simulink model "sedemo_rsim_resource_alloc"  (Simulink 7.5)
settings: Solver=VariableStepDiscrete  StartTime=0.0  StopTime=1000  MaxStep=inf  RelTol=1e-3
PreLoadFcn:
  | TrialPoolSize = 3;
undefined symbols (not defined in the file or in its folder): des_subsystemblock, des_subsysteminport, des_subsystemoutport, des_subsystemsupportblock
libraries: simeventssink1 x4, simeventsrouting1 x4, simeventsgenerators1 x3, simeventsqueue1 x2, simeventstranslate1 x2, simeventsserver1 x2, simeventsentitymanage1 x2, simeventsattributes2 x1, simeventsprobes1 x1, simeventsinfo x1
CloseFcn:
  | clear TrialPoolSize;
settings Model: Creator=The MathWorks Inc.  TunableVars=TrialPoolSize  TunableVarsStorageClass=Auto
settings DataIOCC: SaveOutput=off  SaveTime=off
settings OptimizationCC: InlineParams=on
settings DebuggingCC: AlgebraicLoopMsg=error  SolverPrmCheckMsg=none  StrictBusMsg=Warning
settings HardwareCC: TargetEndianess=LittleEndian  TargetHWDeviceType=MATLAB Host  ProdEqTarget=off
settings RTWCC: SystemTargetFile=rsim.tlc  TemplateMakefile=rsim_default_tmf  Description=Rapid Simulation Target  RTWVerbose=off  ProcessScript=rsim_make_rtw_hook
settings RSimTargetCC: TargetFunctionLibrary=ANSI_C  ERTMultiwordTypeDef=System defined  ERTCodeCoverageTool=None  ERTMultiwordLength=256  IsPILTarget=off  EnableShiftOperators=on  PortableWordSizes=off
settings SimEventsCC: propDiagAttribOutput=1  propDiagFcnCallOutput=1  propDiagStatOutput=0

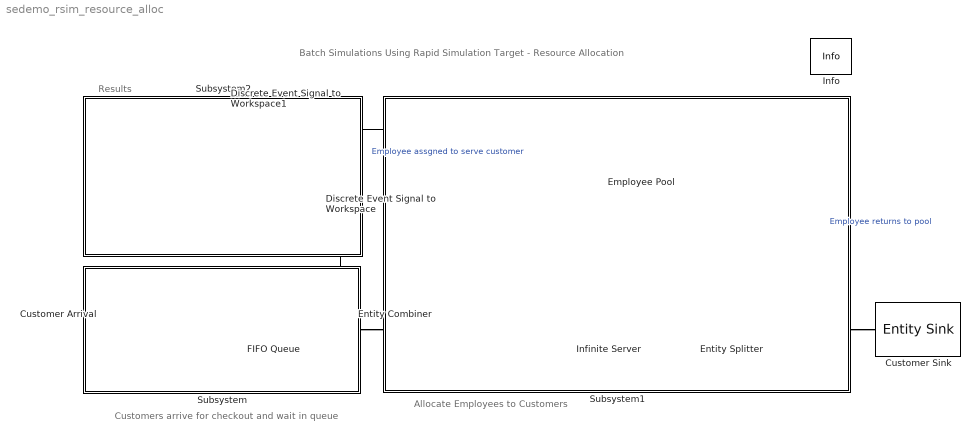
== system sedemo_rsim_resource_alloc ==
  note: Batch Simulations Using Rapid Simulation Target - Resource Allocation
  note: Customers arrive for checkout and wait in queue
  note: Allocate Employees to Customers
  note: Results
  Customer Arrival : Subsystem
  Customer Sink : simeventssink1/Entity Sink  Priority=1  SystemSampleTime=-1  AvailableForArrivals=on  StatNumberArrived=Off
  Discrete Event Signal to Workspace : simeventssink1/Discrete Event Signal to Workspace  SystemSampleTime=-1  VariableName=customer_wait  SaveFormat=Structure With Time  IsMonitorOnly=off  IsRecordIC=off
  Discrete Event Signal to Workspace1 : simeventssink1/Discrete Event Signal to Workspace  SystemSampleTime=-1  VariableName=employee_idle  SaveFormat=Structure With Time  IsMonitorOnly=off  IsRecordIC=off
  Employee Pool : Subsystem  mask{PoolSize=TrialPoolSize}
      mask prompts: PoolSize "Size of Employee Pool"
  Entity Combiner : simeventsentitymanage1/Entity Combiner  Priority=1  SystemSampleTime=-1  NumberInputPorts=2  RetainComponentEntities=on  AttributeAccessibility=on  TimerAccessibility=on  AttributeCopied=on  TimerCopied=on  StatNumberDeparted=Off  EvaluatedNumPorts=2
      settings: AttributesFormatString=Employee assigned to\nserve the customer
  Entity Splitter : simeventsentitymanage1/Entity Splitter  Priority=1  SystemSampleTime=-1  NumberOutputPorts=2  SplitEntityWhen=All entity output ports are not blocked  OutputPortPrecedence=OUT1 port  InitialSeed=56789  ActionUponPortMismatch=Continue  ActionUponBlocking=Discard entity  StatNumberArrived=Off  StatNumberDeparted=Off  EvaluatedNumPorts=2
      settings: AttributesFormatString=Service Completed
  FIFO Queue : simeventsqueue1/FIFO Queue  Priority=1  SystemSampleTime=-1  Capacity=25  EnableTOPort=off  StatNumberDeparted=Off  StatNumberInBlock=Off  StatPendingEntity=Off  StatAverageWait=On  StatAverageQueueLength=Off  StatNumberTimedout=Off
      settings: AttributesFormatString=Customer queue
  Infinite Server : simeventsserver1/Infinite Server  Priority=1  SystemSampleTime=-1  ServiceTimeFrom=Attribute  ServiceTime=1  AttributeName=ServiceTime  PriorityServiceCompletion=500  EnableTOPort=off  StatNumberDeparted=Off  StatNumberInBlock=Off  StatPendingEntity=Off  StatNumberPending=Off  StatAverageWait=Off  StatNumberTimedout=Off
      settings: AttributesFormatString=Employee serves\nthe customer
  Info : simeventsinfo/Info  SystemSampleTime=-1
  Subsystem : Subsystem
      mask Display: disp('')
  Subsystem1 : Subsystem
      mask Display: disp('')
  Subsystem2 : Subsystem
      mask Display: disp('')
  wires:
  FIFO Queue/1 -> Discrete Event Signal to Workspace/1
  Employee Pool/1(idle) -> Discrete Event Signal to Workspace1/1
  connections:
  Customer Arrival/RConn1 -- FIFO Queue/LConn1
  FIFO Queue/RConn1 -- Entity Combiner/LConn2
  Entity Combiner/RConn1 -- Infinite Server/LConn1
  Infinite Server/RConn1 -- Entity Splitter/LConn1
  Entity Splitter/RConn2 -- Customer Sink/LConn1
  Employee Pool/RConn1 -- Entity Combiner/LConn1  "Employee assgned to serve customer"
  Entity Splitter/RConn1 -- Employee Pool/LConn1  "Employee returns to pool"

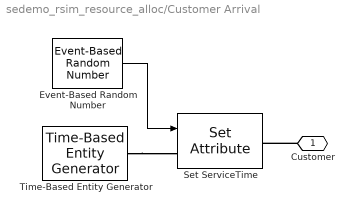
== system sedemo_rsim_resource_alloc/Customer Arrival ==
  Event-Based Random Number : simeventsgenerators1/Signal Generators/Event-Based Random Number  SystemSampleTime=-1  distribution=Uniform  meanExp=2  minUnif=2  maxUnif=10  pOneBern=0.25  pSuccessBino=0.5  numTrialBino=1  meanNorm=0  stdNorm=1  minTri=1  maxTri=3  modeTri=2  thresholdLogn=0  scaleLogn=1  shapeLogn=1  pSuccessGeo=0.5  meanPoiss=1  thresholdLogl=0  scaleLogl=1  thresholdGam=0  scaleGam=1  shapeGam=1  minBeta=0  maxBeta=1  shape1Beta=1  shape2Beta=1  minUnid=0  maxUnid=1  numValueUnid=2  thresholdWbl=0  scaleWbl=1  shapeWbl=1  valueVecCont=[0 1]  cdfVecCont=[0 1]  valueVecDisc=[0 1]  probVecDisc=[0.5 0.5]  seed=6723510  IsProcessed=on  isConnected=1
  Set ServiceTime : simeventsattributes2/Set Attribute  Priority=1  DialogController=des_ddg_create  DialogControllerArgs=DataTag1  SystemSampleTime=-1  AttributeFrom=Signal port  AttributeName=ServiceTime  AttributeTreatAsVector=1  AttributeValue=1  AttributeCreate=on  StatNumberDeparted=Off  EvaluatedAttributeValue={[]}
  Time-Based Entity Generator : simeventsgenerators1/Entity Generators/Time-Based Entity Generator  Priority=1  DialogController=des_ddg_create  DialogControllerArgs=DataTag3  SystemSampleTime=-1  GenerateEntitiesUpon=Intergeneration time from dialog  Distribution=Exponential  Minimum=0  Maximum=1  Mean=1  InitialSeed=6726727  Period=1  PriorityEntityGeneration=300  GenerateEntityAtSimulationStart=on  ResponseWhenBlocked=Pause generation  ResponseWhenUnblocked=Immediate restart  EntityType=Blank  StatNumberDeparted=Off  StatPendingEntity=Off  StatAverageIntergenerationTime=Off
  Customer : PMIOPort  Port=1  Side=Right
  wires:
  Event-Based Random Number/1 -> Set ServiceTime/1
  connections:
  Time-Based Entity Generator/RConn1 -- Set ServiceTime/LConn1
  Customer/RConn1 -- Set ServiceTime/RConn1

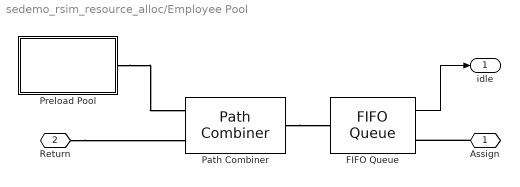
== system sedemo_rsim_resource_alloc/Employee Pool ==
  FIFO Queue : simeventsqueue1/FIFO Queue  Priority=1  SystemSampleTime=-1  Capacity=25  EnableTOPort=off  StatNumberDeparted=Off  StatNumberInBlock=Off  StatPendingEntity=Off  StatAverageWait=On  StatAverageQueueLength=Off  StatNumberTimedout=Off
      settings: AttributesFormatString=Employee Pool
  Path Combiner : simeventsrouting1/Path Combiner  Priority=1  SystemSampleTime=-1  NumberInputPorts=2  InputPortPrecedence=IN1 port  InitialSeed=45675  SpecifyEventPriority=off  PriorityPathCombinerPortPrecedenceSelection=4100  StatNumberDeparted=Off  StatLastArrivalPort=Off  EvaluatedNumPorts=2
  Preload Pool : Subsystem
  Assign : PMIOPort  Port=1  Side=Right
  Return : PMIOPort  Port=2  Side=Left
  idle : Outport
  wires:
  FIFO Queue/1 -> idle/1
  connections:
  Path Combiner/RConn1 -- FIFO Queue/LConn1
  Assign/RConn1 -- FIFO Queue/RConn1
  Return/RConn1 -- Path Combiner/LConn2
  Preload Pool/RConn1 -- Path Combiner/LConn1

== system sedemo_rsim_resource_alloc/Subsystem ==

== system sedemo_rsim_resource_alloc/Subsystem1 ==

== system sedemo_rsim_resource_alloc/Subsystem2 ==

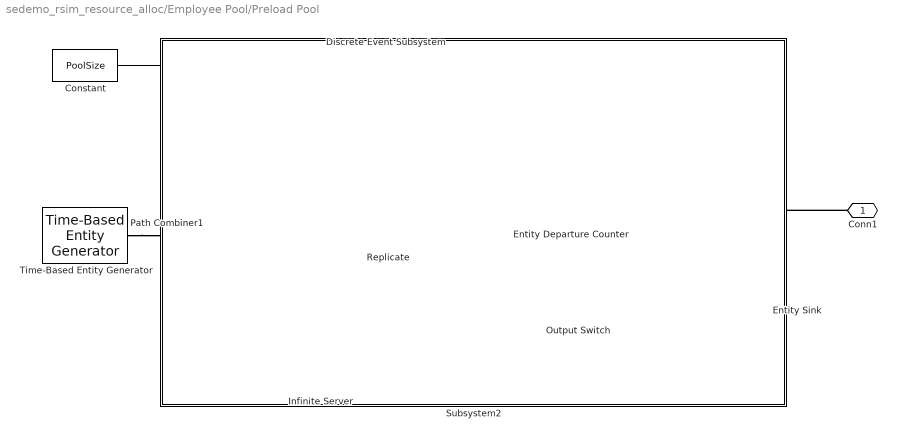
== system sedemo_rsim_resource_alloc/Employee Pool/Preload Pool ==
  Constant : Constant  Value=PoolSize  OutDataType=fixdt(1, 16)  OutScaling=2^0
  Discrete Event Subsystem : Subsystem  LoadFcn=des_subsystemblock(gcb, 'load');  InitFcn=des_subsystemblock(gcb, 'init');  StartFcn=des_subsystemblock(gcb, 'start');  StopFcn=des_subsystemblock(gcb, 'stop');
      settings: CopyFcn=des_subsystemblock(gcb, 'copy');  DeleteFcn=des_subsystemblock(gcb, 'delete');  UndoDeleteFcn=des_subsystemblock(gcb, 'undodelete');  ModelCloseFcn=des_subsystemblock(gcb, 'modelclose');  PreSaveFcn=des_subsystemblock(gcb, 'presave');  NameChangeFcn=des_subsystemblock(gcb, 'namechange');  OpenFcn=des_subsystemblock(gcb, 'open');  ParentCloseFcn=des_subsystemblock(gcb, 'parentclose');  ErrorFcn=des_subsystemerror
      mask Type: Discrete Event Subsystem
      mask Help: helpview(simeventsbhelp);
  Entity Departure Counter : simeventsprobes1/Entity Departure Counter  Priority=1  SystemSampleTime=-1  NumberDepartedToSignal=On  NumberDepartedToAttribute=Off  NumberDepartedAttributeName=Count  CreateAttribute=on  CounterResetTypeOption=Trigger from port tr  CounterResetEdgeOption=Rising  SpecifyEventPriority=on  PriorityEntityCounterReset=1
  Entity Sink : simeventssink1/Entity Sink  Priority=1  SystemSampleTime=-1  AvailableForArrivals=on  StatNumberArrived=Off
  Infinite Server : simeventsserver1/Infinite Server  Priority=1  SystemSampleTime=-1  ServiceTimeFrom=Dialog  ServiceTime=0  AttributeName=ServiceTime  PriorityServiceCompletion=10  EnableTOPort=off  StatNumberDeparted=Off  StatNumberInBlock=Off  StatPendingEntity=Off  StatNumberPending=Off  StatAverageWait=Off  StatNumberTimedout=Off
  Output Switch : simeventsrouting1/Output Switch  Priority=1  SystemSampleTime=-1  NumberOutputPorts=2  SwitchingCriterion=From signal port p  InitialSeed=34567  AttributeName=Attribute1  InitialConditionsOpt=on  InitialConditions=1  EntityBufferOpt=on  SpecifyEventPriority=off  PriorityOutputSwitchSelectPort=4100  TimeoutPortOpt=off  StatNumberDeparted=Off  StatNumberTimedOut=Off  StatPendingEntity=Off  StatLastDeparturePort=Off  EvaluatedNumPorts=2
  Path Combiner1 : simeventsrouting1/Path Combiner  Priority=1  SystemSampleTime=-1  NumberInputPorts=2  InputPortPrecedence=IN1 port  InitialSeed=45675  SpecifyEventPriority=off  PriorityPathCombinerPortPrecedenceSelection=4100  StatNumberDeparted=Off  StatLastArrivalPort=Off  EvaluatedNumPorts=2
  Replicate : simeventsrouting1/Replicate  Priority=1  SystemSampleTime=-1  NumberOutputPorts=2  ReplicateEntityWhen=All entity output ports are not blocked  OutputPortPrecedence=OUT1 port  InitialSeed=56789  ActionUponBlocking=Discard entity  StatNumberArrived=Off  StatNumberDeparted=Off  EvaluatedNumPorts=2
  Subsystem2 : Subsystem
      mask Display: disp('')
  Time-Based Entity Generator : simeventsgenerators1/Entity Generators/Time-Based Entity Generator  Priority=1  DialogController=des_ddg_create  DialogControllerArgs=DataTag24  SystemSampleTime=-1  GenerateEntitiesUpon=Intergeneration time from dialog  Distribution=Constant  Minimum=0  Maximum=1  Mean=2  InitialSeed=6726727  Period=1e5  PriorityEntityGeneration=10  GenerateEntityAtSimulationStart=on  ResponseWhenBlocked=Pause generation  ResponseWhenUnblocked=Immediate restart  EntityType=Blank  StatNumberDeparted=Off  StatPendingEntity=Off  StatAverageIntergenerationTime=Off
  Conn1 : PMIOPort  Port=1  Side=Right
  wires:
  Entity Departure Counter/1 -> Discrete Event Subsystem/2(Din1)
  Discrete Event Subsystem/2(Dout1) -> Entity Departure Counter/1
  Discrete Event Subsystem/1(Dout) -> Output Switch/1
  Constant/1 -> Discrete Event Subsystem/1(Din)
  connections:
  Replicate/RConn1 -- Entity Departure Counter/LConn1
  Output Switch/RConn2 -- Entity Sink/LConn1
  Output Switch/RConn1 -- Infinite Server/LConn1
  Infinite Server/RConn1 -- Path Combiner1/LConn1
  Replicate/RConn2 -- Output Switch/LConn1
  Time-Based Entity Generator/RConn1 -- Path Combiner1/LConn2
  Path Combiner1/RConn1 -- Replicate/LConn1
  Conn1/RConn1 -- Entity Departure Counter/RConn1

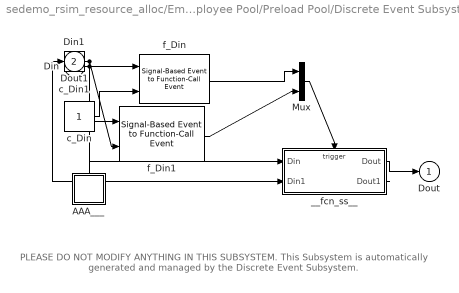
== system sedemo_rsim_resource_alloc/Employee Pool/Preload Pool/Discrete Event Subsystem ==
  note: PLEASE DO NOT MODIFY ANYTHING IN THIS SUBSYSTEM.
      | This Subsystem is automatically generated and
      | managed by the Discrete Event Subsystem.
  Din : Inport  DataType=double  OutDataType=sfix(16)  OutScaling=2^0  OutDataTypeStr=double
  Din1 : Inport  Port=2  DataType=double  OutDataTypeStr=double
  AAA___ : Subsystem  LoadFcn=des_subsystemsupportblock(gcb, 'load');  InitFcn=des_subsystemsupportblock(gcb, 'init');  StartFcn=des_subsystemsupportblock(gcb, 'start');  StopFcn=des_subsystemsupportblock(gcb, 'stop');
      settings: CopyFcn=des_subsystemsupportblock(gcb, 'copy');  DeleteFcn=des_subsystemsupportblock(gcb, 'delete');  UndoDeleteFcn=des_subsystemsupportblock(gcb, 'undodelete');  ModelCloseFcn=des_subsystemsupportblock(gcb, 'modelclose');  PreSaveFcn=des_subsystemsupportblock(gcb, 'presave');  NameChangeFcn=des_subsystemsupportblock(gcb, 'namechange');  OpenFcn=des_subsystemsupportblock(gcb, 'open');  ParentCloseFcn=des_subsystemsupportblock(gcb, 'parentclose');
  Mux : Mux  Inputs=2
  __fcn_ss__ : Subsystem  TreatAsAtomicUnit=on
      settings: PropExecContextOutsideSubsystem=on
  c_Din : Constant  OutDataType=sfix(16)  OutScaling=2^0
  c_Din1 : Constant
  f_Din : simeventstranslate1/Signal-Based Event to Function-Call Event  Priority=1  SystemSampleTime=-1  GenerateFunctionCallUpon=Sample time hit from port ts  SignalEdgeOption=Rising  EnableE1Port=on  EnableF2Port=off  EnableE2Port=off  SpecifyEventPriority=off  PriorityFunctionCall=20  FunctionCallDelayFrom=Dialog  DelayFunctionCall=0  StatNumberF1Calls=Off  StatNumberF2Calls=Off  MaskBlockType=DESS_EVENT_PORT
  f_Din1 : simeventstranslate1/Signal-Based Event to Function-Call Event  Priority=1  SystemSampleTime=-1  GenerateFunctionCallUpon=Sample time hit from port ts  SignalEdgeOption=Rising  EnableE1Port=on  EnableF2Port=off  EnableE2Port=off  SpecifyEventPriority=off  PriorityFunctionCall=20  FunctionCallDelayFrom=Dialog  DelayFunctionCall=0  StatNumberF1Calls=Off  StatNumberF2Calls=Off  MaskBlockType=DESS_EVENT_PORT
  Dout : Outport  OutDataType=sfix(16)  OutScaling=2^0
  Dout1 : Outport  Port=2
  wires:
  __fcn_ss__/1(Dout) -> Dout/1
  f_Din/1 -> Mux/1
  c_Din/1 -> f_Din/2
  Mux/1 -> __fcn_ss__/Trigger
  f_Din1/1 -> Mux/2
  c_Din1/1 -> f_Din1/2
  __fcn_ss__/2(Dout1) -> Dout1/1
  Din/1 -> f_Din/1, __fcn_ss__/1(Din)
  Din1/1 -> f_Din1/1, __fcn_ss__/2(Din1)

== system sedemo_rsim_resource_alloc/Employee Pool/Preload Pool/Subsystem2 ==

== system sedemo_rsim_resource_alloc/Employee Pool/Preload Pool/Discrete Event Subsystem/AAA___ ==

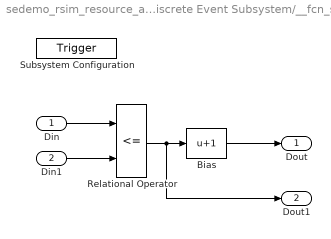
== system sedemo_rsim_resource_alloc/Employee Pool/Preload Pool/Discrete Event Subsystem/__fcn_ss__ ==
  Din : Inport  LoadFcn=des_subsysteminport(gcb, 'load');  InitFcn=des_subsysteminport(gcb, 'init');  StartFcn=des_subsysteminport(gcb, 'start');  StopFcn=des_subsysteminport(gcb, 'stop');  OutDataType=sfix(16)  OutScaling=2^0  mask(Discrete Event Inport){PermitSubsystemEvents=on, TypeOfEvent=Sample time hit, SignalEdgeOption=Rising, SpecifyEventPriority=off, PrioritySubsystemEvent=20}
      mask prompts: PermitSubsystemEvents "Execute subsystem upon signal-based events"; TypeOfEvent "Type of signal-based event:"; SignalEdgeOption "Type of change in signal value:"; SpecifyEventPriority "Resolve simultaneous signal updates according to event priority"; PrioritySubsystemEvent "Event priority:"
      mask help: Input port for a Discrete Event Subsystem block. This block can conditionally execute the subsystem upon signal-based events that meet specified criteria.
      mask init:
      | des_subsystemmask(gcb, 'init','apply')
      settings: CopyFcn=des_subsysteminport(gcb, 'copy');  DeleteFcn=des_subsysteminport(gcb, 'delete');  UndoDeleteFcn=des_subsysteminport(gcb, 'undodelete');  ModelCloseFcn=des_subsysteminport(gcb, 'modelclose');  PreSaveFcn=des_subsysteminport(gcb, 'presave');  NameChangeFcn=des_subsysteminport(gcb, 'namechange');  ParentCloseFcn=des_subsysteminport(gcb, 'parentclose');
      mask Help: helpview(simeventsbhelp);
      mask StyleString: checkbox,popup(Change in signal|Trigger|Sample time hit),popup(Rising|Falling|Either),checkbox,edit
      mask CallbackString: des_subsystemmask(gcb, 'cbPermitSubsystemEvents', 'noapply');|des_subsystemmask(gcb,'cbTypeOfEvent','noapply');||des_subsystemmask(gcb, 'cbSpecifyEventPriority', 'noapply');|
  Din1 : Inport  LoadFcn=des_subsysteminport(gcb, 'load');  InitFcn=des_subsysteminport(gcb, 'init');  StartFcn=des_subsysteminport(gcb, 'start');  StopFcn=des_subsysteminport(gcb, 'stop');  Port=2  OutDataType=sfix(16)  OutScaling=2^0  mask(Discrete Event Inport){PermitSubsystemEvents=on, TypeOfEvent=Sample time hit, SignalEdgeOption=Rising, SpecifyEventPriority=off, PrioritySubsystemEvent=20}
      mask prompts: PermitSubsystemEvents "Execute subsystem upon signal-based events"; TypeOfEvent "Type of signal-based event:"; SignalEdgeOption "Type of change in signal value:"; SpecifyEventPriority "Resolve simultaneous signal updates according to event priority"; PrioritySubsystemEvent "Event priority:"
      mask help: Input port for a Discrete Event Subsystem block. This block can conditionally execute the subsystem upon signal-based events that meet specified criteria.
      mask init:
      | des_subsystemmask(gcb, 'init','apply')
      settings: CopyFcn=des_subsysteminport(gcb, 'copy');  DeleteFcn=des_subsysteminport(gcb, 'delete');  UndoDeleteFcn=des_subsysteminport(gcb, 'undodelete');  ModelCloseFcn=des_subsysteminport(gcb, 'modelclose');  PreSaveFcn=des_subsysteminport(gcb, 'presave');  NameChangeFcn=des_subsysteminport(gcb, 'namechange');  ParentCloseFcn=des_subsysteminport(gcb, 'parentclose');
      mask Help: helpview(simeventsbhelp);
      mask StyleString: checkbox,popup(Change in signal|Trigger|Sample time hit),popup(Rising|Falling|Either),checkbox,edit
      mask CallbackString: des_subsystemmask(gcb, 'cbPermitSubsystemEvents', 'noapply');|des_subsystemmask(gcb,'cbTypeOfEvent','noapply');||des_subsystemmask(gcb, 'cbSpecifyEventPriority', 'noapply');|
  Subsystem Configuration : TriggerPort  TriggerType=function-call
      settings: CopyFcn=des_subsystemconfigblock(gcb, 'copy');  DeleteFcn=des_subsystemconfigblock(gcb, 'delete');  UndoDeleteFcn=des_subsystemconfigblock(gcb, 'undodelete');
      mask Type: Subsystem Configuration
      mask Description: Configuration for a Discrete Event Subsystem block. Every discrete event subsystem window must contain exactly one copy of this configuration block. Do not delete this block.
      mask Help: helpview(simeventsbhelp);
      mask Display: disp('Do Not Delete');
  Bias : Bias  Bias=1
  Relational Operator : RelationalOperator  Operator=<=  LogicOutDataTypeMode=Specify via dialog  LogicDataType=float('double')  OutDataTypeStr=float('double')
  Dout : Outport  LoadFcn=des_subsystemoutport(gcb, 'load');  InitFcn=des_subsystemoutport(gcb, 'init');  StartFcn=des_subsystemoutport(gcb, 'start');  StopFcn=des_subsystemoutport(gcb, 'stop');  OutDataType=sfix(16)  OutScaling=2^0
      settings: CopyFcn=des_subsystemoutport(gcb, 'copy');  DeleteFcn=des_subsystemoutport(gcb, 'delete');  UndoDeleteFcn=des_subsystemoutport(gcb, 'undodelete');  ModelCloseFcn=des_subsystemoutport(gcb, 'modelclose');  PreSaveFcn=des_subsystemoutport(gcb, 'presave');  NameChangeFcn=des_subsystemoutport(gcb, 'namechange');  ParentCloseFcn=des_subsystemoutport(gcb, 'parentclose');
      mask Type: Discrete Event Outport
      mask Description: Provide an output port for a Discrete Event Subsystem block.
      mask Help: helpview(simeventsbhelp);
  Dout1 : Outport  LoadFcn=des_subsystemoutport(gcb, 'load');  InitFcn=des_subsystemoutport(gcb, 'init');  StartFcn=des_subsystemoutport(gcb, 'start');  StopFcn=des_subsystemoutport(gcb, 'stop');  Port=2  OutDataType=sfix(16)  OutScaling=2^0
      settings: CopyFcn=des_subsystemoutport(gcb, 'copy');  DeleteFcn=des_subsystemoutport(gcb, 'delete');  UndoDeleteFcn=des_subsystemoutport(gcb, 'undodelete');  ModelCloseFcn=des_subsystemoutport(gcb, 'modelclose');  PreSaveFcn=des_subsystemoutport(gcb, 'presave');  NameChangeFcn=des_subsystemoutport(gcb, 'namechange');  ParentCloseFcn=des_subsystemoutport(gcb, 'parentclose');
      mask Type: Discrete Event Outport
      mask Description: Provide an output port for a Discrete Event Subsystem block.
      mask Help: helpview(simeventsbhelp);
  wires:
  Din/1 -> Relational Operator/1
  Din1/1 -> Relational Operator/2
  Relational Operator/1 -> Bias/1, Dout1/1
  Bias/1 -> Dout/1
